simulink model "EGAS_throttle"  (R2021b)
settings: Solver=VariableStepAuto  StartTime=0.0  StopTime=10  RelTol=1e-3
model workspace (MAT data in the model file):
  Cs = 3
  Eeq = 0.523598775598
  J = 0.000245
  Sig = Simulink.Signal
  Sig.DataType = 'auto'
  Sig.Dimensions = -1
  Sig.DimensionsMode = 'auto'
  Sig.Complexity = 'auto'
  Sig.SampleTime = -1
  Sig.SamplingMode = 'auto'
  Sig1 = Simulink.Signal
  Sig1.DataType = 'auto'
  Sig1.Dimensions = -1
  Sig1.DimensionsMode = 'auto'
  Sig1.Complexity = 'auto'
  Sig1.SampleTime = -1
  Sig1.SamplingMode = 'auto'
  Sig2 = Simulink.Signal
  Sig2.DataType = 'auto'
  Sig2.Dimensions = -1
  Sig2.DimensionsMode = 'auto'
  Sig2.Complexity = 'auto'
  Sig2.SampleTime = -1
  Sig2.SamplingMode = 'auto'
  Sig3 = Simulink.Signal
  Sig3.DataType = 'auto'
  Sig3.Dimensions = -1
  Sig3.DimensionsMode = 'auto'
  Sig3.Complexity = 'auto'
  Sig3.SampleTime = -1
  Sig3.SamplingMode = 'auto'
  Sig4 = Simulink.Signal
  Sig4.DataType = 'auto'
  Sig4.Dimensions = -1
  Sig4.DimensionsMode = 'auto'
  Sig4.Complexity = 'auto'
  Sig4.SampleTime = -1
  Sig4.SamplingMode = 'auto'
  Sig5 = Simulink.Signal
  Sig5.DataType = 'auto'
  Sig5.Dimensions = -1
  Sig5.DimensionsMode = 'auto'
  Sig5.Complexity = 'auto'
  Sig5.SampleTime = -1
  Sig5.SamplingMode = 'auto'
  Ts = 0.01
  kd = 0.03
  ki = 0.3
  kp = 0.2
  ks = 0.02
libraries: simulink x1
settings Model: Creator=student  LastModifiedBy=Lenovo
settings SolverCC: AlgebraicLoopSolver=TrustRegion
settings DataIOCC: ReturnWorkspaceOutputs=off
settings DebuggingCC: SFMachineParentedDataDiag=warning  ArithmeticOperatorsInVariantConditions=warning
settings SFSimCC: CustomCodeUndefinedFunction=UseInterfaceOnly

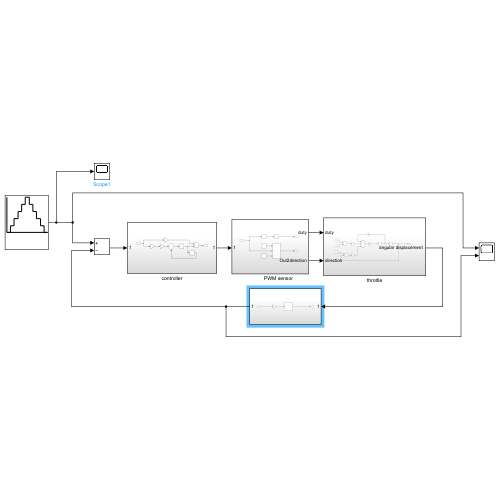
[thumbnail: Simulink's stored preview of the top-level diagram]
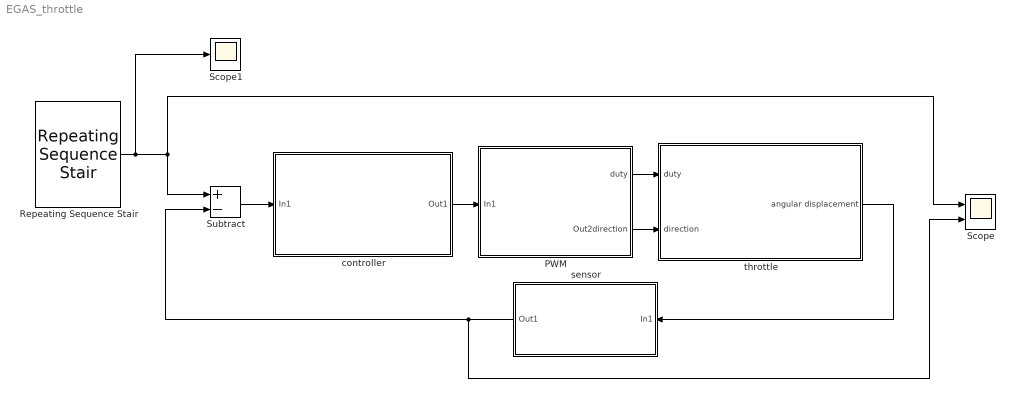
== system EGAS_throttle ==
  PWM : Subsystem
  Repeating Sequence Stair : simulink/Sources/Repeating Sequence Stair  OutValues=[0 1 2 3 4 5 4 3 2 1 0].'  tsamp=-1  OutMin=[]  OutMax=[]  OutDataTypeStr=double  OutputDataTypeScalingMode=double  OutDataType=fixdt(0,8)  ConRadixGroup=Best Precision: Vector-wise  OutScaling=2^-12
  Scope : Scope  NumInputPorts=2
  Scope1 : Scope
  Subtract : Sum  Inputs=+-
  "controller " : Subsystem
  "sensor " : Subsystem
  "throttle " : Subsystem
  wires:
  "controller "/1(Out1) -> PWM/1(In1)
  Subtract/1 -> "controller "/1(In1)
  "sensor "/1(Out1) -> Scope/2, Subtract/2
  Repeating Sequence Stair/1 -> Scope1/1, Subtract/1, Scope/1
  "throttle "/1("angular displacement ") -> "sensor "/1(In1)
  PWM/1(duty) -> "throttle "/1(duty)
  PWM/2(Out2direction) -> "throttle "/2("direction ")

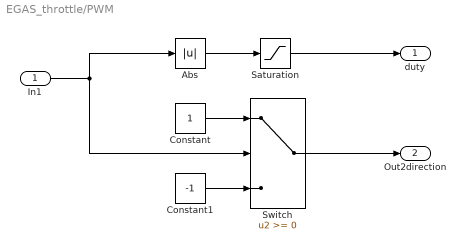
== system EGAS_throttle/PWM ==
  In1 : Inport
  Abs : Abs
  Constant : Constant
  Constant1 : Constant  Value=-1
  Saturation : Saturate  UpperLimit=1  LowerLimit=0
  Switch : Switch
  duty : Outport  VectorParamsAs1DForOutWhenUnconnected=off
  Out2direction : Outport  Port=2  VectorParamsAs1DForOutWhenUnconnected=off
  wires:
  Switch/1 -> Out2direction/1
  In1/1 -> Switch/2, Abs/1
  Constant1/1 -> Switch/3
  Abs/1 -> Saturation/1
  Constant/1 -> Switch/1
  Saturation/1 -> duty/1

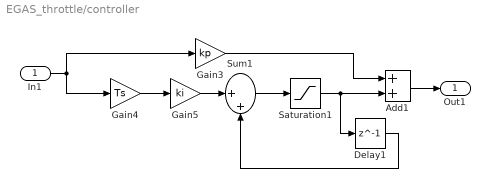
== system EGAS_throttle/controller  ==
  In1 : Inport
  Add1 : Sum
  Delay1 : Delay  DelayLength=1
  Gain3 : Gain  Gain=kp
  Gain4 : Gain  Gain=Ts
  Gain5 : Gain  Gain=ki
  Saturation1 : Saturate  UpperLimit=1  LowerLimit=-1
  Sum1 : Sum  Inputs=|++
  Out1 : Outport  VectorParamsAs1DForOutWhenUnconnected=off
  wires:
  Sum1/1 -> Saturation1/1
  Delay1/1 -> Sum1/2
  In1/1 -> Gain3/1, Gain4/1
  Gain5/1 -> Sum1/1
  Saturation1/1 -> Delay1/1, Add1/2
  Gain3/1 -> Add1/1
  Add1/1 -> Out1/1
  Gain4/1 -> Gain5/1

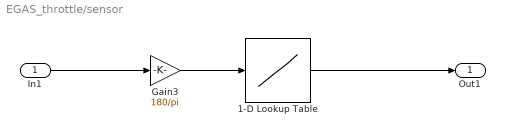
== system EGAS_throttle/sensor  ==
  In1 : Inport
  1-D Lookup Table : Lookup_n-D  NumberOfTableDimensions=1  BreakpointsForDimension1=[0 90]  Table=[0.5 4.5]  InternalRulePriority=Speed  RndMeth=Simplest  InputSameDT=on
  Gain3 : Gain  Gain=180/pi
  Out1 : Outport  VectorParamsAs1DForOutWhenUnconnected=off
  wires:
  In1/1 -> Gain3/1
  Gain3/1 -> 1-D Lookup Table/1
  1-D Lookup Table/1 -> Out1/1

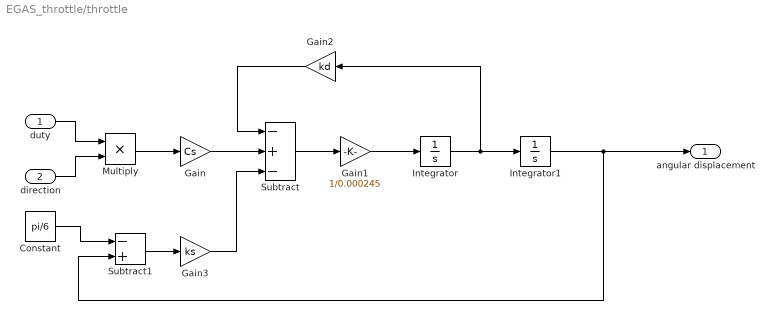
== system EGAS_throttle/throttle  ==
  duty : Inport
  "direction " : Inport  Port=2
  Constant : Constant  Value=pi/6
  Gain : Gain  Gain=Cs
  Gain1 : Gain  Gain=1/0.000245
  Gain2 : Gain  Gain=kd
  Gain3 : Gain  Gain=ks
  Integrator : Integrator
  Integrator1 : Integrator  LimitOutput=on  UpperSaturationLimit=90  LowerSaturationLimit=0
  Multiply : Product
  Subtract : Sum  Inputs=-+-
  Subtract1 : Sum  Inputs=-+
  "angular displacement " : Outport  VectorParamsAs1DForOutWhenUnconnected=off
  wires:
  Constant/1 -> Subtract1/1
  Multiply/1 -> Gain/1
  Integrator/1 -> Integrator1/1, Gain2/1
  Gain2/1 -> Subtract/1
  Gain3/1 -> Subtract/3
  Subtract1/1 -> Gain3/1
  "direction "/1 -> Multiply/2
  duty/1 -> Multiply/1
  Gain/1 -> Subtract/2
  Gain1/1 -> Integrator/1
  Subtract/1 -> Gain1/1
  Integrator1/1 -> Subtract1/2, "angular displacement "/1
